simulink model "tank2"  (R2020b)
settings: Solver=VariableStepAuto  StartTime=0.0  StopTime=40000  RelTol=1e-3
values from neighbouring files (symbols this model uses):
  a_out = 0    [TankFillingScript.m]
  c = 16    [TankFillingScript.m]
  k_out = 0.1587/60    (= 0.002645)    [TankFillingScript.m]
settings Model: Creator=StevensUser  LastModifiedBy=mreiff

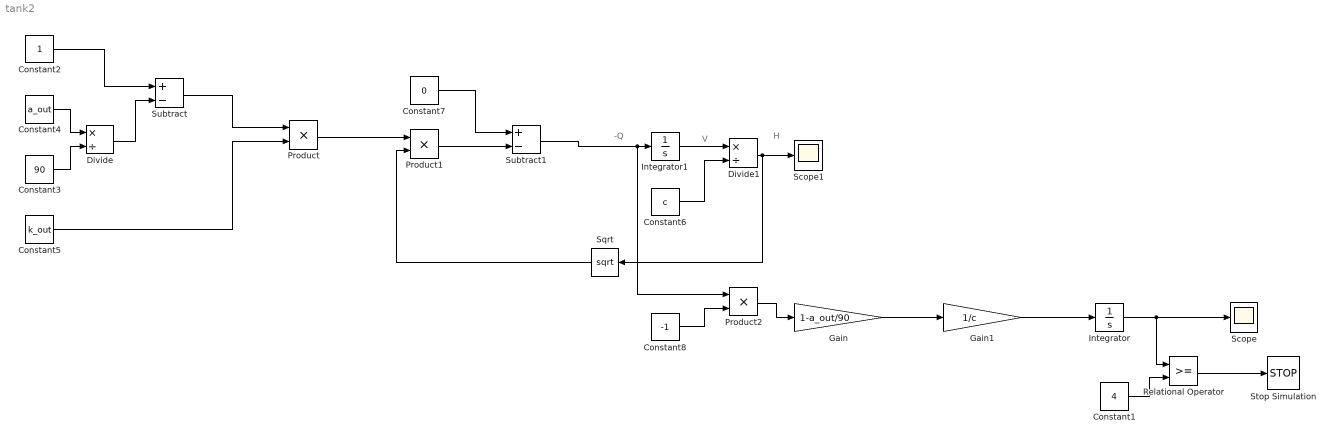
== system tank2 ==
  note: V
  note: -Q
  note: H
  Constant1 : Constant  Value=4
  Constant2 : Constant
  Constant3 : Constant  Value=90
  Constant4 : Constant  Value=a_out
  Constant5 : Constant  Value=k_out
  Constant6 : Constant  Value=c
  Constant7 : Constant  Value=0
  Constant8 : Constant  Value=-1
  Divide : Product  Inputs=*/
  Divide1 : Product  Inputs=*/
  Gain : Gain  Gain=1-a_out/90
  Gain1 : Gain  Gain=1/c
  Integrator : Integrator
  Integrator1 : Integrator  InitialCondition=64
  Product : Product
  Product1 : Product
  Product2 : Product
  Relational Operator : RelationalOperator  OutDataTypeStr=boolean  RndMeth=Simplest
  Scope : Scope
  Scope1 : Scope
  Sqrt : Sqrt  SaturateOnIntegerOverflow=on
  Stop Simulation : Stop
  Subtract : Sum  Inputs=+-
  Subtract1 : Sum  Inputs=+-
  wires:
  Gain/1 -> Gain1/1
  Gain1/1 -> Integrator/1
  Relational Operator/1 -> Stop Simulation/1
  Constant1/1 -> Relational Operator/2
  Integrator/1 -> Relational Operator/1, Scope/1
  Constant6/1 -> Divide1/2
  Integrator1/1 -> Divide1/1
  Constant4/1 -> Divide/1
  Product/1 -> Product1/1
  Divide/1 -> Subtract/2
  Constant3/1 -> Divide/2
  Divide1/1 -> Sqrt/1, Scope1/1
  Subtract/1 -> Product/1
  Constant2/1 -> Subtract/1
  Constant5/1 -> Product/2
  Sqrt/1 -> Product1/2
  Product1/1 -> Subtract1/2
  Subtract1/1 -> Product2/1, Integrator1/1
  Constant7/1 -> Subtract1/1
  Constant8/1 -> Product2/2
  Product2/1 -> Gain/1
